simulink model "IEEE5BusSystemModel_std_UFLS"  (R2019b)
settings: Solver=ode4  StartTime=0.0  StopTime=300  MaxStep=1e-4  RelTol=1e-3
InitFcn:
  | startup_RTS
values from neighbouring files (symbols this model uses):
  C = b/(2*pi*60*Zn)    [startup_RTS.m]
  C0 = C/3    [startup_RTS.m]
  fn = 50    [startup_RTS.m]
  In = Sn/(sqrt(3)*Vn)    [startup_RTS.m]
  L = x*Zn/(2*pi*60)    [startup_RTS.m]
  L0 = 3*L    [startup_RTS.m]
  len = ceil(0.95*300000*T_prop)    [startup_RTS.m]
  PL1 = 300e6    (= 300000000)    [startup_RTS.m]
  PL2 = 300e6    (= 300000000)    [startup_RTS.m]
  PL3 = 300e6    (= 300000000)    [startup_RTS.m]
  QL1 = 30e6    (= 30000000)    [startup_RTS.m]
  QL2 = 30e6    (= 30000000)    [startup_RTS.m]
  QL3 = 30e6    (= 30000000)    [startup_RTS.m]
  R = r*Zn    [startup_RTS.m]
  R0 = 3*R    [startup_RTS.m]
  Sn = 1000e6    (= 1000000000)    [startup_RTS.m]
  t_cont = 100    [startup_RTS.m]
  Vn = 345e3    (= 345000)    [startup_RTS.m]
undefined symbols (not defined in the file or in its folder): D1, Delta
libraries: powerlib x42, powerlib_meascontrol x39, dspswit3 x10, dspstat3 x3, sps_avr x3, spsExcitationSystemModel x3
(part 2 of 7)

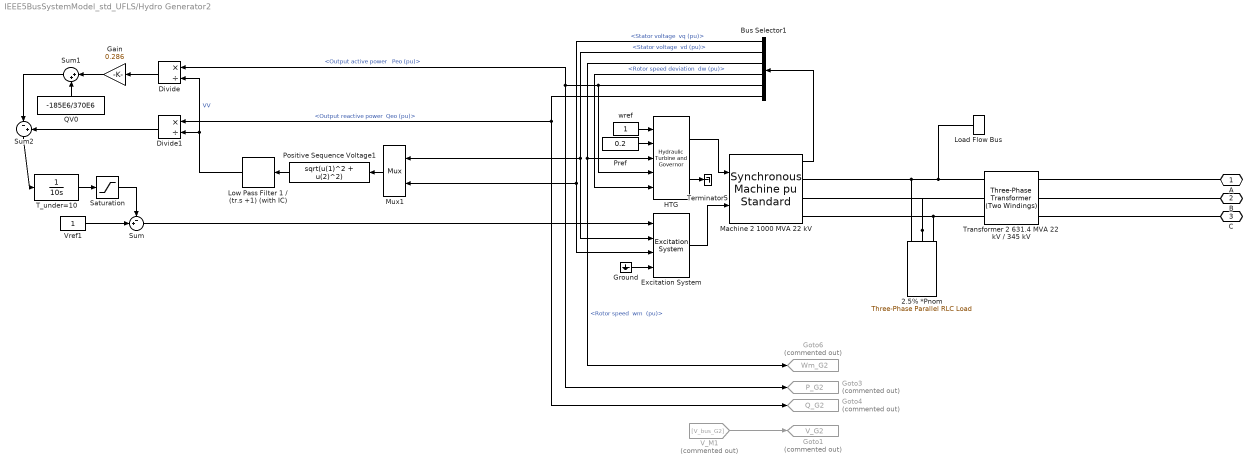
== system IEEE5BusSystemModel_std_UFLS/Hydro Generator2 ==
  2.5% *Pnom : powerlib/Elements/Three-Phase Parallel RLC Load  LConnTagsString=A|B|C  Configuration=Y (grounded)  NominalVoltage=vNom*1e3  Vabc=[1e3 1e3 1e3]  Vabcp=[1e3 1e3 1e3]  NominalFrequency=50  UnbalancedPower=off  ActivePower=pTotal*1e6*0.025  InductivePower=0  CapacitivePower=0  Pabc=[10e3 9e3 11e3]  QLabc=[100 90 110]  QCabc=[100 90 110]  Pabcp=[10e3 9e3 11e3]  QLabcp=[100 90 110]  QCabcp=[100 90 110]  Measurements=None  LoadType=constant Z
      settings: SourceProductName=Simscape Electrical
  Bus Selector1 : BusSelector  OutputSignals="dq0 components.Stator voltage  vq (pu),dq0 components.Stator voltage  vd (pu),Mechanical.Rotor speed  wm  (pu),Mechanical.Rotor speed deviation  dw (pu),Output active power   Peo (pu),Output reactive power  Qeo (pu)"
  Divide : Product  Inputs=*/
  Divide1 : Product  Inputs=*/
  Excitation System : sps_avr/Excitation System  tr=20e-3  reg=[ 200, 0.02 ]  exc=[ 1, 0 .19]  tgr=[ 0, 0 ]  damp=[ 0.0012, 1 ]  sat=[ 0, 0 ]  lim=[ 0, 7.32, 0 ]  v0=[1 1.0103]
      settings: SourceProductName=Simscape Electrical  SourceProductBaseCode=PS
  Gain : Gain  Gain=0.286
  Goto1 : Goto  Commented=on  GotoTag=V_G2  TagVisibility=global
  Goto3 : Goto  Commented=on  GotoTag=P_G2  TagVisibility=global
  Goto4 : Goto  Commented=on  GotoTag=Q_G2  TagVisibility=global
  Goto6 : Goto  Commented=on  GotoTag=Wm_G2  TagVisibility=global
  Ground : Ground
  HTG : powerlib/Machines/Hydraulic Turbine and Governor  sm="[ 10/3  0.07 ]"  gate="[  0.01  0.97518  -0.1  0.1 ]"  reg="[  0.05  1.163  0.105  0  0.01  ]"  hyd="[  0  2.67  ]"  dref=0  po=0.2002
      settings: SourceProductName=Simscape Electrical  SourceProductBaseCode=PS
  Load Flow Bus : powerlib/Measurements/Load Flow Bus  LConnTagsString=a  Phases=single  Connectors=on one side  ID=BUS_2_3  Vbase=22e3  Vref=1  Vangle=0  VLF=1  VLFb=1  VLFc=1  angleLF=-4.793  angleLFb=0  angleLFc=0
      settings: SourceProductName=Simscape Electrical
  Low Pass Filter 1 / (tr.s +1) (with IC) : spsExcitationSystemModel/Discrete/Low Pass Filter 1 // (tr.s +1) (with IC)  FilterType=Lowpass  Tc=20e-3  Ts=25e-6  Initialize=on  Vac_Init=[0 0 50]  Vdc_Init=1  PlotResponse=off  param1=[1 500 0.1]
      settings: SourceProductName=Simscape Electrical  SourceProductBaseCode=PS
  Machine 2 1000 MVA 22 kV : powerlib/Machines/Synchronous Machine pu Standard  PresetModel=No  MechanicalLoad=Mechanical power Pm  ShowDetailedParameters=on  RotorType=Round  Units=per unit standard parameters  MeasurementBus=off  NominalParameters=[pTotal*1e+006 vNom*1e3 fNom]  Reactances1=[ 1.693 0.4 0.2 1.618 0.967 0.2 0.035 ]  Reactances2=[1.699 0.174 0.109 0.838 0.185 0.069]  dAxisTimeConstants=Open-circuit  qAxisTimeConstants=Open-circuit  TimeConstants1=[]  TimeConstants2=[6.56 0.03 1.5 0.04]  TimeConstants3=[]  TimeConstants4=[]  TimeConstants5=[ 9.2, 0.01, 0.01 ]  TimeConstants6=[]  TimeConstants7=[0.024 0.006 0.006]  TimeConstants8=[1 2 3 1]  StatorResistance=0.005  Mechanical=[5.28 0.02558 2]  PolePairs=2  InitialConditions=[0 -76.0492 0.202092 0.202092 0.202092 3.45918 -116.541 123.459 1.01026]  SetSaturation=off  Saturation=[0.6404,0.7127,0.8441,0.9214,0.9956,1.082,1.19,1.316,1.457;0.7,0.7698,0.8872,0.9466,0.9969,1.046,1.1,1.151,1.201]  LoadFlowParameters=[1 524200000 21604 0]  TsPowergui=0  TsBlock=-1  IterativeModel=Trapezoidal non iterative  IterativeDiscreteModel=Trapezoidal non iterative  BusType=PV  Pref=200e6  Qref=0  Qmin=-100e6  Qmax=100e6  PLF=0  QLF=0
      settings: AttributesFormatString=\n\n  SourceProductName=Simscape Electrical
  Mux1 : Mux  Inputs=2
  Positive Sequence Voltage1 : Fcn  Expr=sqrt(u(1)^2 + u(2)^2)
  Pref : Constant  Value=0.2
  QV0 : Constant  Value=-185E6/370E6
  Saturation : Saturate  UpperLimit=0  LowerLimit=-10
  Sum : Sum  Inputs=-+|
  Sum1 : Sum  Inputs=|++
  Sum2 : Sum  Inputs=|-+
  T_under=10 : TransferFcn  Denominator=[10 0 ]
  Terminator5 : Terminator
  Transformer 2 631.4 MVA 22 kV / 345 kV : powerlib/Elements/Three-Phase Transformer (Two Windings)  Winding1Connection=Delta (D1)  Winding2Connection=Yg  CoreType=Three single-phase transformers  SetSaturation=off  Hysteresis=off  DataFile='hysteresis'  SetInitialFlux=off  Measurements=None  UNITS=pu  NominalPower=[ pTotal*1e+6 fNom ]  Winding1="[vNom*1e3   0.0     0.025*pTotal/100/2]"  Winding2="[ 1.07*345e3  0.0     0.025*pTotal/100/2 ]"  Rm=500  Lm=500  L0=0.5  Saturation="[ 0,0  ;  0.005,1.2  ;  1.0,1.4 ]"  InitialFluxes=[ 0.8 , -0.8 , 0.7 ]  BreakLoop=off  DiscreteSolver=Trapezoidal iterative  DataType=off  TransfoNumber=0
      settings: SourceProductName=Simscape Electrical
  V_M1 : From  Commented=on  GotoTag=V_bus_G2
  Vref1 : Constant
  wref : Constant
  A : PMIOPort  Side=Right
  B : PMIOPort  Port=2  Side=Right
  C : PMIOPort  Port=3  Side=Right
  wires:
  Ground/1 -> Excitation System/4
  HTG/2 -> Terminator5/1
  Sum/1 -> Excitation System/1
  Pref/1 -> HTG/2
  wref/1 -> HTG/1
  Excitation System/1 -> Machine 2 1000 MVA 22 kV/2
  HTG/1 -> Machine 2 1000 MVA 22 kV/1
  Machine 2 1000 MVA 22 kV/1 -> Bus Selector1/1
  Bus Selector1/3 -> HTG/3, Goto6/1  "<Rotor speed  wm  (pu)>"
  Bus Selector1/4 -> HTG/5  "<Rotor speed deviation  dw (pu)>"
  Bus Selector1/6 -> Divide1/1, Goto4/1  "<Output reactive power  Qeo (pu)>"
  V_M1/1 -> Goto1/1
  Saturation/1 -> Sum/1
  Gain/1 -> Sum1/1
  Sum1/1 -> Sum2/1
  Positive Sequence Voltage1/1 -> Low Pass Filter 1 / (tr.s +1) (with IC)/1
  Vref1/1 -> Sum/2
  Bus Selector1/5 -> HTG/4, Divide/1, Goto3/1  "<Output active power   Peo (pu)>"
  Divide/1 -> Gain/1
  Low Pass Filter 1 / (tr.s +1) (with IC)/1 -> Divide1/2, Divide/2  "VV"
  QV0/1 -> Sum1/2
  Sum2/1 -> T_under=10/1
  T_under=10/1 -> Saturation/1
  Mux1/1 -> Positive Sequence Voltage1/1
  Divide1/1 -> Sum2/2
  Bus Selector1/1 -> Mux1/2, Excitation System/3  "<Stator voltage  vq (pu)>"
  Bus Selector1/2 -> Mux1/1, Excitation System/2  "<Stator voltage  vd (pu)>"
  connections:
  C/RConn1 -- Transformer 2 631.4 MVA 22 kV / 345 kV/RConn3
  Transformer 2 631.4 MVA 22 kV / 345 kV/LConn1 -- Load Flow Bus/LConn1 -- Machine 2 1000 MVA 22 kV/RConn1 -- 2.5% *Pnom/LConn1
  2.5% *Pnom/LConn2 -- Transformer 2 631.4 MVA 22 kV / 345 kV/LConn2 -- Machine 2 1000 MVA 22 kV/RConn2
  A/RConn1 -- Transformer 2 631.4 MVA 22 kV / 345 kV/RConn1
  B/RConn1 -- Transformer 2 631.4 MVA 22 kV / 345 kV/RConn2
  Machine 2 1000 MVA 22 kV/RConn3 -- Transformer 2 631.4 MVA 22 kV / 345 kV/LConn3 -- 2.5% *Pnom/LConn3

== system IEEE5BusSystemModel_std_UFLS/Subsystem ==
  f1 : Inport
  f2 : Inport  Port=2
  f3 : Inport  Port=3
  Enable : EnablePort  PropagateVarSize=During execution
  Gain : Gain  Gain=fn
  Gain1 : Gain  Gain=fn
  Gain2 : Gain  Gain=fn
  loadshedding : Subsystem  TreatAsAtomicUnit=on  SystemSampleTime=0.0025
  loadshedding1 : Subsystem  TreatAsAtomicUnit=on  SystemSampleTime=0.0025
  loadshedding2 : Subsystem  TreatAsAtomicUnit=on  SystemSampleTime=0.0025
  Shedding factor 1 : Outport  VectorParamsAs1DForOutWhenUnconnected=off
  Shedding factor 2 : Outport  Port=2  VectorParamsAs1DForOutWhenUnconnected=off
  Shedding factor 3 : Outport  Port=3  VectorParamsAs1DForOutWhenUnconnected=off
  wires:
  Gain2/1 -> loadshedding2/1(Freq)
  loadshedding/1(Shedding factor) -> Shedding factor 1/1
  f1/1 -> Gain/1
  f3/1 -> Gain2/1
  Gain/1 -> loadshedding/1(Freq)
  Gain1/1 -> loadshedding1/1(Freq)
  f2/1 -> Gain1/1
  loadshedding1/1(Shedding factor) -> Shedding factor 2/1
  loadshedding2/1(Shedding factor) -> Shedding factor 3/1

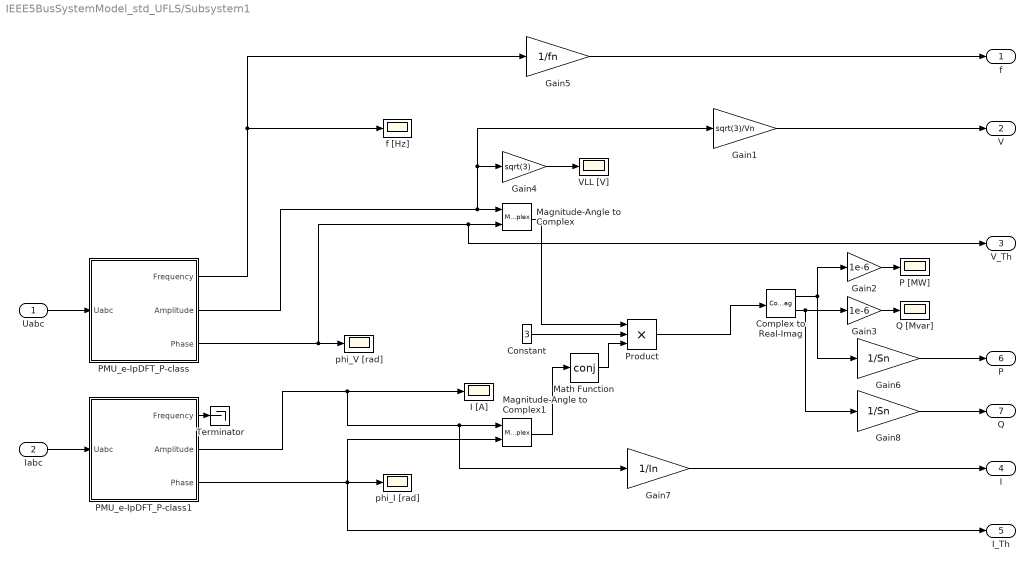
== system IEEE5BusSystemModel_std_UFLS/Subsystem1 ==
  Uabc : Inport  OutDataTypeStr=double  PortDimensions=3  SampleTime=[5.0000000000000002e-05,0]
  Iabc : Inport  Port=2  OutDataTypeStr=double  PortDimensions=3  SampleTime=[5.0000000000000002e-05,0]
  Complex to Real-Imag : ComplexToRealImag
  Constant : Constant  Value=3
  Gain1 : Gain  Gain=sqrt(3)/Vn
  Gain2 : Gain  Gain=1e-6
  Gain3 : Gain  Gain=1e-6
  Gain4 : Gain  Gain=sqrt(3)
  Gain5 : Gain  Gain=1/fn
  Gain6 : Gain  Gain=1/Sn
  Gain7 : Gain  Gain=1/In
  Gain8 : Gain  Gain=1/Sn
  I [A] : Scope
  Magnitude-Angle to Complex : MagnitudeAngleToComplex
  Magnitude-Angle to Complex1 : MagnitudeAngleToComplex
  Math Function : Math  Operator=conj  SaturateOnIntegerOverflow=on
  P [MW] : Scope
  PMU_e-IpDFT_P-class : Subsystem  TreatAsAtomicUnit=on  SystemSampleTime=100e-6  mask{f0=50, Fr=50, Fs=1e4, T=0.06, enable_comp=off, TdF=10}
      mask prompts: f0 "Nominal frequency (Hz)"; Fr "Data reporting rate (frames/s)"; Fs "Sampling rate (Hz)"; T "Window length (s)"; enable_comp "Compensate clock drift"; TdF "Clock drift measurement window length (s)"
      mask init:
      | dF = 1/T;
      | M = round(T*Fs);
      | kmax = round (f0*T);
      | k = kmax-2:kmax+2;
      | Wk = exp(-1i*2*pi*k./M);
      | Tr = 1/Fr;
      | Ts_p=1/Fs;
      mask DialogControl ParameterTabVar0 Prompt: Settings
  PMU_e-IpDFT_P-class1 : Subsystem  TreatAsAtomicUnit=on  SystemSampleTime=100e-6  mask{f0=50, Fr=50, Fs=1e4, T=0.06, enable_comp=off, TdF=10}
      mask prompts: f0 "Nominal frequency (Hz)"; Fr "Data reporting rate (frames/s)"; Fs "Sampling rate (Hz)"; T "Window length (s)"; enable_comp "Compensate clock drift"; TdF "Clock drift measurement window length (s)"
      mask init:
      | dF = 1/T;
      | M = round(T*Fs);
      | kmax = round (f0*T);
      | k = kmax-2:kmax+2;
      | Wk = exp(-1i*2*pi*k./M);
      | Tr = 1/Fr;
      | Ts_p=1/Fs;
      mask DialogControl ParameterTabVar0 Prompt: Settings
  Product : Product  Inputs=3
  Q [Mvar] : Scope
  Terminator : Terminator
  VLL [V] : Scope
  f [Hz] : Scope
  phi_I [rad] : Scope
  phi_V [rad] : Scope
  f : Outport  OutDataTypeStr=double  PortDimensions=1  SampleTime=[0.02,0]  VectorParamsAs1DForOutWhenUnconnected=off
  V : Outport  Port=2  OutDataTypeStr=double  PortDimensions=1  SampleTime=[0.02,0]  VectorParamsAs1DForOutWhenUnconnected=off
  V_Th : Outport  Port=3  OutDataTypeStr=double  PortDimensions=1  SampleTime=[0.02,0]  VectorParamsAs1DForOutWhenUnconnected=off
  I : Outport  Port=4  OutDataTypeStr=double  PortDimensions=1  SampleTime=[0.02,0]  VectorParamsAs1DForOutWhenUnconnected=off
  I_Th : Outport  Port=5  OutDataTypeStr=double  PortDimensions=1  SampleTime=[0.02,0]  VectorParamsAs1DForOutWhenUnconnected=off
  P : Outport  Port=6  OutDataTypeStr=double  PortDimensions=1  SampleTime=[0.02,0]  VectorParamsAs1DForOutWhenUnconnected=off
  Q : Outport  Port=7  OutDataTypeStr=double  PortDimensions=1  SampleTime=[0.02,0]  VectorParamsAs1DForOutWhenUnconnected=off
  wires:
  Gain8/1 -> Q/1
  Gain7/1 -> I/1
  Gain5/1 -> f/1
  Gain6/1 -> P/1
  Complex to Real-Imag/2 -> Gain3/1, Gain8/1
  Complex to Real-Imag/1 -> Gain2/1, Gain6/1
  Product/1 -> Complex to Real-Imag/1
  Math Function/1 -> Product/3
  Constant/1 -> Product/2
  Magnitude-Angle to Complex1/1 -> Math Function/1
  Gain1/1 -> V/1
  Magnitude-Angle to Complex/1 -> Product/1
  PMU_e-IpDFT_P-class1/1(Frequency) -> Terminator/1
  Gain4/1 -> VLL [V]/1
  Gain3/1 -> Q [Mvar]/1
  Uabc/1 -> PMU_e-IpDFT_P-class/1(Uabc)
  PMU_e-IpDFT_P-class1/2(Amplitude) -> I [A]/1, Magnitude-Angle to Complex1/1, Gain7/1
  PMU_e-IpDFT_P-class1/3(Phase) -> Magnitude-Angle to Complex1/2, phi_I [rad]/1, I_Th/1
  Gain2/1 -> P [MW]/1
  PMU_e-IpDFT_P-class/1(Frequency) -> f [Hz]/1, Gain5/1
  PMU_e-IpDFT_P-class/2(Amplitude) -> Magnitude-Angle to Complex/1, Gain4/1, Gain1/1
  PMU_e-IpDFT_P-class/3(Phase) -> Magnitude-Angle to Complex/2, V_Th/1, phi_V [rad]/1
  Iabc/1 -> PMU_e-IpDFT_P-class1/1(Uabc)

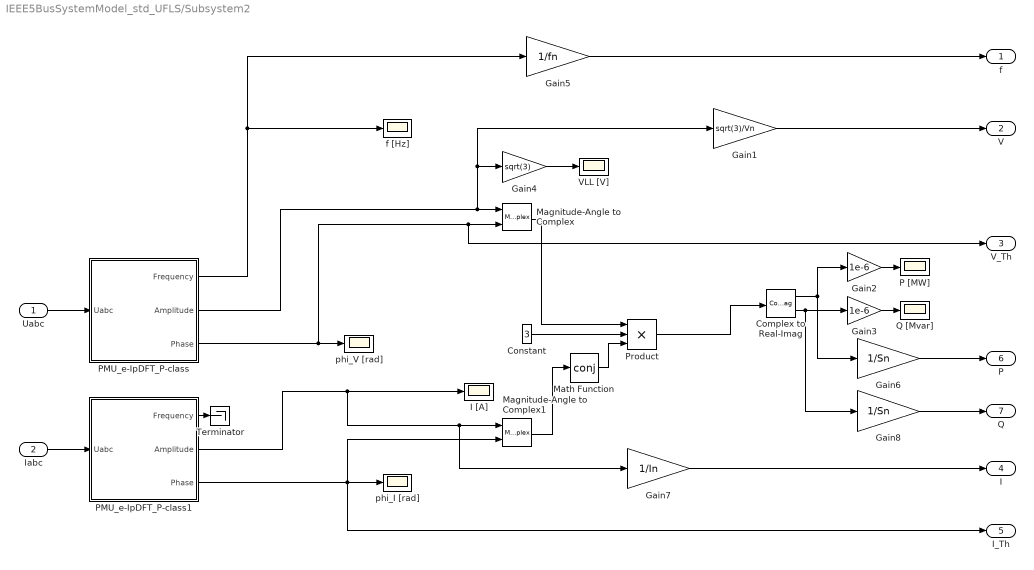
== system IEEE5BusSystemModel_std_UFLS/Subsystem2 ==
  Uabc : Inport  OutDataTypeStr=double  PortDimensions=3  SampleTime=[5.0000000000000002e-05,0]
  Iabc : Inport  Port=2  OutDataTypeStr=double  PortDimensions=3  SampleTime=[5.0000000000000002e-05,0]
  Complex to Real-Imag : ComplexToRealImag
  Constant : Constant  Value=3
  Gain1 : Gain  Gain=sqrt(3)/Vn
  Gain2 : Gain  Gain=1e-6
  Gain3 : Gain  Gain=1e-6
  Gain4 : Gain  Gain=sqrt(3)
  Gain5 : Gain  Gain=1/fn
  Gain6 : Gain  Gain=1/Sn
  Gain7 : Gain  Gain=1/In
  Gain8 : Gain  Gain=1/Sn
  I [A] : Scope
  Magnitude-Angle to Complex : MagnitudeAngleToComplex
  Magnitude-Angle to Complex1 : MagnitudeAngleToComplex
  Math Function : Math  Operator=conj  SaturateOnIntegerOverflow=on
  P [MW] : Scope
  PMU_e-IpDFT_P-class : Subsystem  TreatAsAtomicUnit=on  SystemSampleTime=100e-6  mask{f0=50, Fr=50, Fs=1e4, T=0.06, enable_comp=off, TdF=10}
      mask prompts: f0 "Nominal frequency (Hz)"; Fr "Data reporting rate (frames/s)"; Fs "Sampling rate (Hz)"; T "Window length (s)"; enable_comp "Compensate clock drift"; TdF "Clock drift measurement window length (s)"
      mask init:
      | dF = 1/T;
      | M = round(T*Fs);
      | kmax = round (f0*T);
      | k = kmax-2:kmax+2;
      | Wk = exp(-1i*2*pi*k./M);
      | Tr = 1/Fr;
      | Ts_p=1/Fs;
      mask DialogControl ParameterTabVar0 Prompt: Settings
  PMU_e-IpDFT_P-class1 : Subsystem  TreatAsAtomicUnit=on  SystemSampleTime=100e-6  mask{f0=50, Fr=50, Fs=1e4, T=0.06, enable_comp=off, TdF=10}
      mask prompts: f0 "Nominal frequency (Hz)"; Fr "Data reporting rate (frames/s)"; Fs "Sampling rate (Hz)"; T "Window length (s)"; enable_comp "Compensate clock drift"; TdF "Clock drift measurement window length (s)"
      mask init:
      | dF = 1/T;
      | M = round(T*Fs);
      | kmax = round (f0*T);
      | k = kmax-2:kmax+2;
      | Wk = exp(-1i*2*pi*k./M);
      | Tr = 1/Fr;
      | Ts_p=1/Fs;
      mask DialogControl ParameterTabVar0 Prompt: Settings
  Product : Product  Inputs=3
  Q [Mvar] : Scope
  Terminator : Terminator
  VLL [V] : Scope
  f [Hz] : Scope
  phi_I [rad] : Scope
  phi_V [rad] : Scope
  f : Outport  OutDataTypeStr=double  PortDimensions=1  SampleTime=[0.02,0]  VectorParamsAs1DForOutWhenUnconnected=off
  V : Outport  Port=2  OutDataTypeStr=double  PortDimensions=1  SampleTime=[0.02,0]  VectorParamsAs1DForOutWhenUnconnected=off
  V_Th : Outport  Port=3  OutDataTypeStr=double  PortDimensions=1  SampleTime=[0.02,0]  VectorParamsAs1DForOutWhenUnconnected=off
  I : Outport  Port=4  OutDataTypeStr=double  PortDimensions=1  SampleTime=[0.02,0]  VectorParamsAs1DForOutWhenUnconnected=off
  I_Th : Outport  Port=5  OutDataTypeStr=double  PortDimensions=1  SampleTime=[0.02,0]  VectorParamsAs1DForOutWhenUnconnected=off
  P : Outport  Port=6  OutDataTypeStr=double  PortDimensions=1  SampleTime=[0.02,0]  VectorParamsAs1DForOutWhenUnconnected=off
  Q : Outport  Port=7  OutDataTypeStr=double  PortDimensions=1  SampleTime=[0.02,0]  VectorParamsAs1DForOutWhenUnconnected=off
  wires:
  Iabc/1 -> PMU_e-IpDFT_P-class1/1(Uabc)
  PMU_e-IpDFT_P-class/3(Phase) -> phi_V [rad]/1, V_Th/1, Magnitude-Angle to Complex/2
  PMU_e-IpDFT_P-class/2(Amplitude) -> Gain1/1, Gain4/1, Magnitude-Angle to Complex/1
  PMU_e-IpDFT_P-class/1(Frequency) -> Gain5/1, f [Hz]/1
  Gain2/1 -> P [MW]/1
  PMU_e-IpDFT_P-class1/3(Phase) -> I_Th/1, phi_I [rad]/1, Magnitude-Angle to Complex1/2
  PMU_e-IpDFT_P-class1/2(Amplitude) -> Gain7/1, Magnitude-Angle to Complex1/1, I [A]/1
  Uabc/1 -> PMU_e-IpDFT_P-class/1(Uabc)
  Gain3/1 -> Q [Mvar]/1
  Gain4/1 -> VLL [V]/1
  PMU_e-IpDFT_P-class1/1(Frequency) -> Terminator/1
  Magnitude-Angle to Complex/1 -> Product/1
  Gain1/1 -> V/1
  Magnitude-Angle to Complex1/1 -> Math Function/1
  Constant/1 -> Product/2
  Math Function/1 -> Product/3
  Product/1 -> Complex to Real-Imag/1
  Complex to Real-Imag/1 -> Gain6/1, Gain2/1
  Complex to Real-Imag/2 -> Gain8/1, Gain3/1
  Gain6/1 -> P/1
  Gain5/1 -> f/1
  Gain7/1 -> I/1
  Gain8/1 -> Q/1

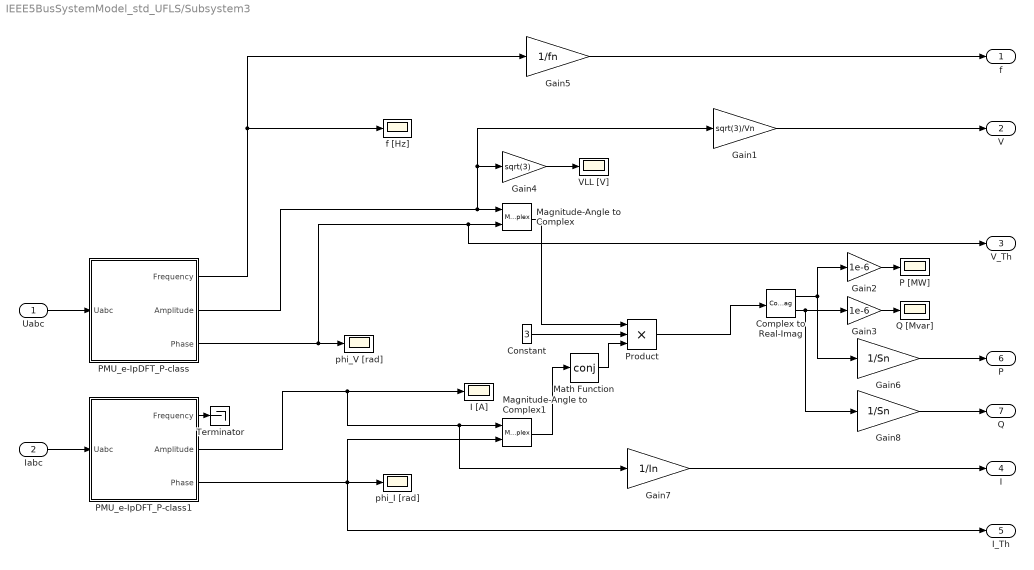
== system IEEE5BusSystemModel_std_UFLS/Subsystem3 ==
  Uabc : Inport  OutDataTypeStr=double  PortDimensions=3  SampleTime=[5.0000000000000002e-05,0]
  Iabc : Inport  Port=2  OutDataTypeStr=double  PortDimensions=3  SampleTime=[5.0000000000000002e-05,0]
  Complex to Real-Imag : ComplexToRealImag
  Constant : Constant  Value=3
  Gain1 : Gain  Gain=sqrt(3)/Vn
  Gain2 : Gain  Gain=1e-6
  Gain3 : Gain  Gain=1e-6
  Gain4 : Gain  Gain=sqrt(3)
  Gain5 : Gain  Gain=1/fn
  Gain6 : Gain  Gain=1/Sn
  Gain7 : Gain  Gain=1/In
  Gain8 : Gain  Gain=1/Sn
  I [A] : Scope
  Magnitude-Angle to Complex : MagnitudeAngleToComplex
  Magnitude-Angle to Complex1 : MagnitudeAngleToComplex
  Math Function : Math  Operator=conj  SaturateOnIntegerOverflow=on
  P [MW] : Scope
  PMU_e-IpDFT_P-class : Subsystem  TreatAsAtomicUnit=on  SystemSampleTime=100e-6  mask{f0=50, Fr=50, Fs=1e4, T=0.06, enable_comp=off, TdF=10}
      mask prompts: f0 "Nominal frequency (Hz)"; Fr "Data reporting rate (frames/s)"; Fs "Sampling rate (Hz)"; T "Window length (s)"; enable_comp "Compensate clock drift"; TdF "Clock drift measurement window length (s)"
      mask init:
      | dF = 1/T;
      | M = round(T*Fs);
      | kmax = round (f0*T);
      | k = kmax-2:kmax+2;
      | Wk = exp(-1i*2*pi*k./M);
      | Tr = 1/Fr;
      | Ts_p=1/Fs;
      mask DialogControl ParameterTabVar0 Prompt: Settings
  PMU_e-IpDFT_P-class1 : Subsystem  TreatAsAtomicUnit=on  SystemSampleTime=100e-6  mask{f0=50, Fr=50, Fs=1e4, T=0.06, enable_comp=off, TdF=10}
      mask prompts: f0 "Nominal frequency (Hz)"; Fr "Data reporting rate (frames/s)"; Fs "Sampling rate (Hz)"; T "Window length (s)"; enable_comp "Compensate clock drift"; TdF "Clock drift measurement window length (s)"
      mask init:
      | dF = 1/T;
      | M = round(T*Fs);
      | kmax = round (f0*T);
      | k = kmax-2:kmax+2;
      | Wk = exp(-1i*2*pi*k./M);
      | Tr = 1/Fr;
      | Ts_p=1/Fs;
      mask DialogControl ParameterTabVar0 Prompt: Settings
  Product : Product  Inputs=3
  Q [Mvar] : Scope
  Terminator : Terminator
  VLL [V] : Scope
  f [Hz] : Scope
  phi_I [rad] : Scope
  phi_V [rad] : Scope
  f : Outport  OutDataTypeStr=double  PortDimensions=1  SampleTime=[0.02,0]  VectorParamsAs1DForOutWhenUnconnected=off
  V : Outport  Port=2  OutDataTypeStr=double  PortDimensions=1  SampleTime=[0.02,0]  VectorParamsAs1DForOutWhenUnconnected=off
  V_Th : Outport  Port=3  OutDataTypeStr=double  PortDimensions=1  SampleTime=[0.02,0]  VectorParamsAs1DForOutWhenUnconnected=off
  I : Outport  Port=4  OutDataTypeStr=double  PortDimensions=1  SampleTime=[0.02,0]  VectorParamsAs1DForOutWhenUnconnected=off
  I_Th : Outport  Port=5  OutDataTypeStr=double  PortDimensions=1  SampleTime=[0.02,0]  VectorParamsAs1DForOutWhenUnconnected=off
  P : Outport  Port=6  OutDataTypeStr=double  PortDimensions=1  SampleTime=[0.02,0]  VectorParamsAs1DForOutWhenUnconnected=off
  Q : Outport  Port=7  OutDataTypeStr=double  PortDimensions=1  SampleTime=[0.02,0]  VectorParamsAs1DForOutWhenUnconnected=off
  wires:
  Gain8/1 -> Q/1
  Gain7/1 -> I/1
  Gain5/1 -> f/1
  Gain6/1 -> P/1
  Complex to Real-Imag/2 -> Gain3/1, Gain8/1
  Complex to Real-Imag/1 -> Gain2/1, Gain6/1
  Product/1 -> Complex to Real-Imag/1
  Math Function/1 -> Product/3
  Constant/1 -> Product/2
  Magnitude-Angle to Complex1/1 -> Math Function/1
  Gain1/1 -> V/1
  Magnitude-Angle to Complex/1 -> Product/1
  PMU_e-IpDFT_P-class1/1(Frequency) -> Terminator/1
  Gain4/1 -> VLL [V]/1
  Gain3/1 -> Q [Mvar]/1
  Uabc/1 -> PMU_e-IpDFT_P-class/1(Uabc)
  PMU_e-IpDFT_P-class1/2(Amplitude) -> I [A]/1, Magnitude-Angle to Complex1/1, Gain7/1
  PMU_e-IpDFT_P-class1/3(Phase) -> Magnitude-Angle to Complex1/2, phi_I [rad]/1, I_Th/1
  Gain2/1 -> P [MW]/1
  PMU_e-IpDFT_P-class/1(Frequency) -> f [Hz]/1, Gain5/1
  PMU_e-IpDFT_P-class/2(Amplitude) -> Magnitude-Angle to Complex/1, Gain4/1, Gain1/1
  PMU_e-IpDFT_P-class/3(Phase) -> Magnitude-Angle to Complex/2, V_Th/1, phi_V [rad]/1
  Iabc/1 -> PMU_e-IpDFT_P-class1/1(Uabc)

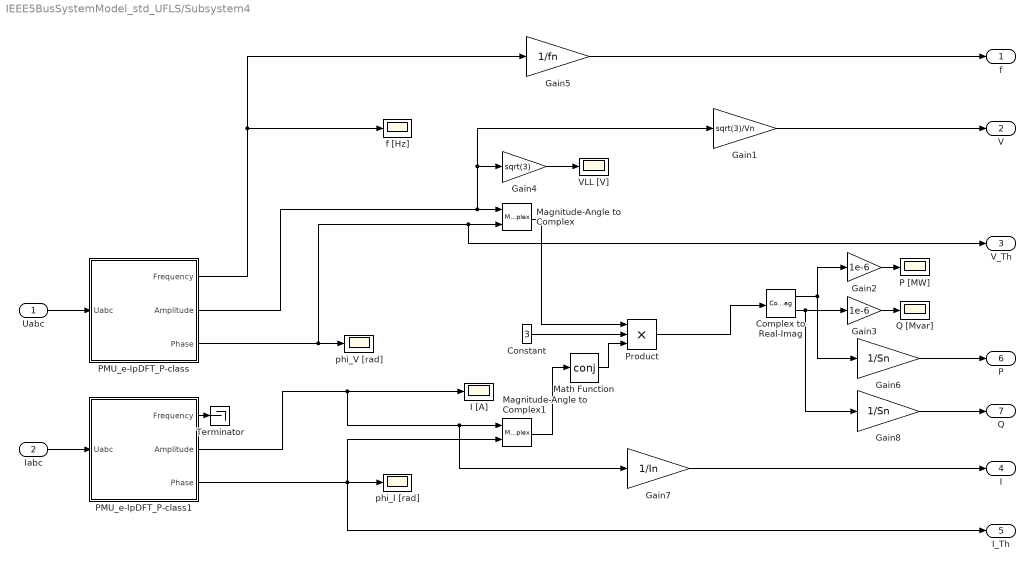
== system IEEE5BusSystemModel_std_UFLS/Subsystem4 ==
  Uabc : Inport  OutDataTypeStr=double  PortDimensions=3  SampleTime=[5.0000000000000002e-05,0]
  Iabc : Inport  Port=2  OutDataTypeStr=double  PortDimensions=3  SampleTime=[5.0000000000000002e-05,0]
  Complex to Real-Imag : ComplexToRealImag
  Constant : Constant  Value=3
  Gain1 : Gain  Gain=sqrt(3)/Vn
  Gain2 : Gain  Gain=1e-6
  Gain3 : Gain  Gain=1e-6
  Gain4 : Gain  Gain=sqrt(3)
  Gain5 : Gain  Gain=1/fn
  Gain6 : Gain  Gain=1/Sn
  Gain7 : Gain  Gain=1/In
  Gain8 : Gain  Gain=1/Sn
  I [A] : Scope
  Magnitude-Angle to Complex : MagnitudeAngleToComplex
  Magnitude-Angle to Complex1 : MagnitudeAngleToComplex
  Math Function : Math  Operator=conj  SaturateOnIntegerOverflow=on
  P [MW] : Scope
  PMU_e-IpDFT_P-class : Subsystem  TreatAsAtomicUnit=on  SystemSampleTime=100e-6  mask{f0=50, Fr=50, Fs=1e4, T=0.06, enable_comp=off, TdF=10}
      mask prompts: f0 "Nominal frequency (Hz)"; Fr "Data reporting rate (frames/s)"; Fs "Sampling rate (Hz)"; T "Window length (s)"; enable_comp "Compensate clock drift"; TdF "Clock drift measurement window length (s)"
      mask init:
      | dF = 1/T;
      | M = round(T*Fs);
      | kmax = round (f0*T);
      | k = kmax-2:kmax+2;
      | Wk = exp(-1i*2*pi*k./M);
      | Tr = 1/Fr;
      | Ts_p=1/Fs;
      mask DialogControl ParameterTabVar0 Prompt: Settings
  PMU_e-IpDFT_P-class1 : Subsystem  TreatAsAtomicUnit=on  SystemSampleTime=100e-6  mask{f0=50, Fr=50, Fs=1e4, T=0.06, enable_comp=off, TdF=10}
      mask prompts: f0 "Nominal frequency (Hz)"; Fr "Data reporting rate (frames/s)"; Fs "Sampling rate (Hz)"; T "Window length (s)"; enable_comp "Compensate clock drift"; TdF "Clock drift measurement window length (s)"
      mask init:
      | dF = 1/T;
      | M = round(T*Fs);
      | kmax = round (f0*T);
      | k = kmax-2:kmax+2;
      | Wk = exp(-1i*2*pi*k./M);
      | Tr = 1/Fr;
      | Ts_p=1/Fs;
      mask DialogControl ParameterTabVar0 Prompt: Settings
  Product : Product  Inputs=3
  Q [Mvar] : Scope
  Terminator : Terminator
  VLL [V] : Scope
  f [Hz] : Scope
  phi_I [rad] : Scope
  phi_V [rad] : Scope
  f : Outport  OutDataTypeStr=double  PortDimensions=1  SampleTime=[0.02,0]  VectorParamsAs1DForOutWhenUnconnected=off
  V : Outport  Port=2  OutDataTypeStr=double  PortDimensions=1  SampleTime=[0.02,0]  VectorParamsAs1DForOutWhenUnconnected=off
  V_Th : Outport  Port=3  OutDataTypeStr=double  PortDimensions=1  SampleTime=[0.02,0]  VectorParamsAs1DForOutWhenUnconnected=off
  I : Outport  Port=4  OutDataTypeStr=double  PortDimensions=1  SampleTime=[0.02,0]  VectorParamsAs1DForOutWhenUnconnected=off
  I_Th : Outport  Port=5  OutDataTypeStr=double  PortDimensions=1  SampleTime=[0.02,0]  VectorParamsAs1DForOutWhenUnconnected=off
  P : Outport  Port=6  OutDataTypeStr=double  PortDimensions=1  SampleTime=[0.02,0]  VectorParamsAs1DForOutWhenUnconnected=off
  Q : Outport  Port=7  OutDataTypeStr=double  PortDimensions=1  SampleTime=[0.02,0]  VectorParamsAs1DForOutWhenUnconnected=off
  wires:
  Iabc/1 -> PMU_e-IpDFT_P-class1/1(Uabc)
  PMU_e-IpDFT_P-class/3(Phase) -> phi_V [rad]/1, V_Th/1, Magnitude-Angle to Complex/2
  PMU_e-IpDFT_P-class/2(Amplitude) -> Gain1/1, Gain4/1, Magnitude-Angle to Complex/1
  PMU_e-IpDFT_P-class/1(Frequency) -> Gain5/1, f [Hz]/1
  Gain2/1 -> P [MW]/1
  PMU_e-IpDFT_P-class1/3(Phase) -> I_Th/1, phi_I [rad]/1, Magnitude-Angle to Complex1/2
  PMU_e-IpDFT_P-class1/2(Amplitude) -> Gain7/1, Magnitude-Angle to Complex1/1, I [A]/1
  Uabc/1 -> PMU_e-IpDFT_P-class/1(Uabc)
  Gain3/1 -> Q [Mvar]/1
  Gain4/1 -> VLL [V]/1
  PMU_e-IpDFT_P-class1/1(Frequency) -> Terminator/1
  Magnitude-Angle to Complex/1 -> Product/1
  Gain1/1 -> V/1
  Magnitude-Angle to Complex1/1 -> Math Function/1
  Constant/1 -> Product/2
  Math Function/1 -> Product/3
  Product/1 -> Complex to Real-Imag/1
  Complex to Real-Imag/1 -> Gain6/1, Gain2/1
  Complex to Real-Imag/2 -> Gain8/1, Gain3/1
  Gain6/1 -> P/1
  Gain5/1 -> f/1
  Gain7/1 -> I/1
  Gain8/1 -> Q/1

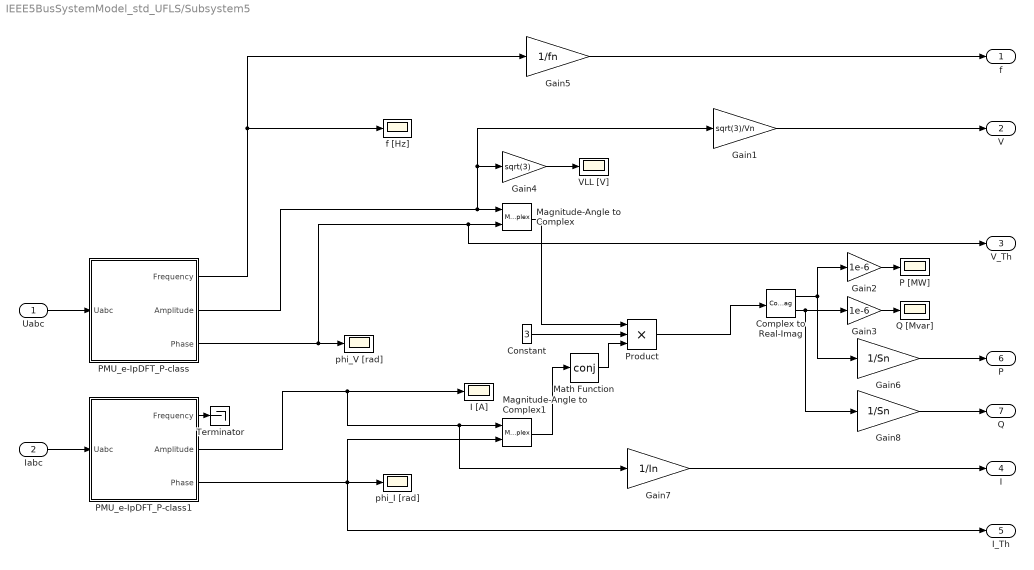
== system IEEE5BusSystemModel_std_UFLS/Subsystem5 ==
  Uabc : Inport  OutDataTypeStr=double  PortDimensions=3  SampleTime=[5.0000000000000002e-05,0]
  Iabc : Inport  Port=2  OutDataTypeStr=double  PortDimensions=3  SampleTime=[5.0000000000000002e-05,0]
  Complex to Real-Imag : ComplexToRealImag
  Constant : Constant  Value=3
  Gain1 : Gain  Gain=sqrt(3)/Vn
  Gain2 : Gain  Gain=1e-6
  Gain3 : Gain  Gain=1e-6
  Gain4 : Gain  Gain=sqrt(3)
  Gain5 : Gain  Gain=1/fn
  Gain6 : Gain  Gain=1/Sn
  Gain7 : Gain  Gain=1/In
  Gain8 : Gain  Gain=1/Sn
  I [A] : Scope
  Magnitude-Angle to Complex : MagnitudeAngleToComplex
  Magnitude-Angle to Complex1 : MagnitudeAngleToComplex
  Math Function : Math  Operator=conj  SaturateOnIntegerOverflow=on
  P [MW] : Scope
  PMU_e-IpDFT_P-class : Subsystem  TreatAsAtomicUnit=on  SystemSampleTime=100e-6  mask{f0=50, Fr=50, Fs=1e4, T=0.06, enable_comp=off, TdF=10}
      mask prompts: f0 "Nominal frequency (Hz)"; Fr "Data reporting rate (frames/s)"; Fs "Sampling rate (Hz)"; T "Window length (s)"; enable_comp "Compensate clock drift"; TdF "Clock drift measurement window length (s)"
      mask init:
      | dF = 1/T;
      | M = round(T*Fs);
      | kmax = round (f0*T);
      | k = kmax-2:kmax+2;
      | Wk = exp(-1i*2*pi*k./M);
      | Tr = 1/Fr;
      | Ts_p=1/Fs;
      mask DialogControl ParameterTabVar0 Prompt: Settings
  PMU_e-IpDFT_P-class1 : Subsystem  TreatAsAtomicUnit=on  SystemSampleTime=100e-6  mask{f0=50, Fr=50, Fs=1e4, T=0.06, enable_comp=off, TdF=10}
      mask prompts: f0 "Nominal frequency (Hz)"; Fr "Data reporting rate (frames/s)"; Fs "Sampling rate (Hz)"; T "Window length (s)"; enable_comp "Compensate clock drift"; TdF "Clock drift measurement window length (s)"
      mask init:
      | dF = 1/T;
      | M = round(T*Fs);
      | kmax = round (f0*T);
      | k = kmax-2:kmax+2;
      | Wk = exp(-1i*2*pi*k./M);
      | Tr = 1/Fr;
      | Ts_p=1/Fs;
      mask DialogControl ParameterTabVar0 Prompt: Settings
  Product : Product  Inputs=3
  Q [Mvar] : Scope
  Terminator : Terminator
  VLL [V] : Scope
  f [Hz] : Scope
  phi_I [rad] : Scope
  phi_V [rad] : Scope
  f : Outport  OutDataTypeStr=double  PortDimensions=1  SampleTime=[0.02,0]  VectorParamsAs1DForOutWhenUnconnected=off
  V : Outport  Port=2  OutDataTypeStr=double  PortDimensions=1  SampleTime=[0.02,0]  VectorParamsAs1DForOutWhenUnconnected=off
  V_Th : Outport  Port=3  OutDataTypeStr=double  PortDimensions=1  SampleTime=[0.02,0]  VectorParamsAs1DForOutWhenUnconnected=off
  I : Outport  Port=4  OutDataTypeStr=double  PortDimensions=1  SampleTime=[0.02,0]  VectorParamsAs1DForOutWhenUnconnected=off
  I_Th : Outport  Port=5  OutDataTypeStr=double  PortDimensions=1  SampleTime=[0.02,0]  VectorParamsAs1DForOutWhenUnconnected=off
  P : Outport  Port=6  OutDataTypeStr=double  PortDimensions=1  SampleTime=[0.02,0]  VectorParamsAs1DForOutWhenUnconnected=off
  Q : Outport  Port=7  OutDataTypeStr=double  PortDimensions=1  SampleTime=[0.02,0]  VectorParamsAs1DForOutWhenUnconnected=off
  wires:
  Iabc/1 -> PMU_e-IpDFT_P-class1/1(Uabc)
  PMU_e-IpDFT_P-class/3(Phase) -> phi_V [rad]/1, V_Th/1, Magnitude-Angle to Complex/2
  PMU_e-IpDFT_P-class/2(Amplitude) -> Gain1/1, Gain4/1, Magnitude-Angle to Complex/1
  PMU_e-IpDFT_P-class/1(Frequency) -> Gain5/1, f [Hz]/1
  Gain2/1 -> P [MW]/1
  PMU_e-IpDFT_P-class1/3(Phase) -> I_Th/1, phi_I [rad]/1, Magnitude-Angle to Complex1/2
  PMU_e-IpDFT_P-class1/2(Amplitude) -> Gain7/1, Magnitude-Angle to Complex1/1, I [A]/1
  Uabc/1 -> PMU_e-IpDFT_P-class/1(Uabc)
  Gain3/1 -> Q [Mvar]/1
  Gain4/1 -> VLL [V]/1
  PMU_e-IpDFT_P-class1/1(Frequency) -> Terminator/1
  Magnitude-Angle to Complex/1 -> Product/1
  Gain1/1 -> V/1
  Magnitude-Angle to Complex1/1 -> Math Function/1
  Constant/1 -> Product/2
  Math Function/1 -> Product/3
  Product/1 -> Complex to Real-Imag/1
  Complex to Real-Imag/1 -> Gain6/1, Gain2/1
  Complex to Real-Imag/2 -> Gain8/1, Gain3/1
  Gain6/1 -> P/1
  Gain5/1 -> f/1
  Gain7/1 -> I/1
  Gain8/1 -> Q/1

== system IEEE5BusSystemModel_std_UFLS/Dynamic Load/Load 8 ==
  note: 200ms buffer for average voltag and frequency
      | to avoid oscillation
  Vabc : Inport
  "[P0,Q0]" : Inport  Port=2
  Buffer1 : Buffer  N=2400  V=2200
  Buffer2 : Buffer  N=240  V=220
  Demux : Demux  Outputs=[1 1 1]
  Gain : Gain  Gain=1/240
  Load shedding : Subsystem  TreatAsAtomicUnit=on  SystemSampleTime=20e-3
  PLL : powerlib_meascontrol/PLL/PLL  Fmin=45  Par_Init=[0, 50]  ParK=[180, 3200, 1]  TcD=1e-3  MaxRateChangeFreq=25  FilterCutOffFreq=25  Ts=1000e-6  AGC=on
      settings: SourceProductName=Simscape Electrical  SourceProductBaseCode=PS
  RMS : dspstat3/RMS  run=off  directionMode=Each column  dimension=1  InputProcessing=Columns as channels (frame based)  reset_popup=None
  Rate Transition : RateTransition  Integrity=off  Deterministic=off  OutPortSampleTime=100e-6
  Rate Transition1 : RateTransition  Integrity=off  Deterministic=off  OutPortSampleTime=100e-6
  Sum of Elements : Sum  Inputs=+
  Terminator : Terminator
  Terminator1 : Terminator
  Terminator2 : Terminator
  Unbuffer : Unbuffer
  Unbuffer1 : Unbuffer
  Load Power : Outport  VectorParamsAs1DForOutWhenUnconnected=off
  wires:
  Load shedding/1(Load Power) -> Load Power/1
  Vabc/1 -> Demux/1
  "[P0,Q0]"/1 -> Load shedding/3(load)
  Buffer1/1 -> RMS/1
  RMS/1 -> Unbuffer/1
  PLL/2 -> Terminator/1
  Unbuffer/1 -> Load shedding/2(Vamp_rms)
  Demux/3 -> Terminator1/1
  Demux/2 -> Terminator2/1
  Demux/1 -> Rate Transition1/1, Rate Transition/1
  PLL/1 -> Buffer2/1
  Buffer2/1 -> Sum of Elements/1
  Sum of Elements/1 -> Gain/1
  Gain/1 -> Unbuffer1/1
  Unbuffer1/1 -> Load shedding/1(" f_PLL")
  Rate Transition/1 -> Buffer1/1
  Rate Transition1/1 -> PLL/1

== system IEEE5BusSystemModel_std_UFLS/Dynamic Load1/Load 8 ==
  note: 200ms buffer for average voltag and frequency
      | to avoid oscillation
  Vabc : Inport
  "[P0,Q0]" : Inport  Port=2
  Buffer1 : Buffer  N=2400  V=2200
  Buffer2 : Buffer  N=240  V=220
  Demux : Demux  Outputs=[1 1 1]
  Gain : Gain  Gain=1/240
  Load shedding : Subsystem  TreatAsAtomicUnit=on  SystemSampleTime=20e-3
  PLL : powerlib_meascontrol/PLL/PLL  Fmin=45  Par_Init=[0, 50]  ParK=[180, 3200, 1]  TcD=1e-3  MaxRateChangeFreq=25  FilterCutOffFreq=25  Ts=1000e-6  AGC=on
      settings: SourceProductName=Simscape Electrical  SourceProductBaseCode=PS
  RMS : dspstat3/RMS  run=off  directionMode=Each column  dimension=1  InputProcessing=Columns as channels (frame based)  reset_popup=None
  Rate Transition : RateTransition  Integrity=off  Deterministic=off  OutPortSampleTime=100e-6
  Rate Transition1 : RateTransition  Integrity=off  Deterministic=off  OutPortSampleTime=100e-6
  Sum of Elements : Sum  Inputs=+
  Terminator : Terminator
  Terminator1 : Terminator
  Terminator2 : Terminator
  Unbuffer : Unbuffer
  Unbuffer1 : Unbuffer
  Load Power : Outport  VectorParamsAs1DForOutWhenUnconnected=off
  wires:
  Rate Transition1/1 -> PLL/1
  Rate Transition/1 -> Buffer1/1
  Unbuffer1/1 -> Load shedding/1(" f_PLL")
  Gain/1 -> Unbuffer1/1
  Sum of Elements/1 -> Gain/1
  Buffer2/1 -> Sum of Elements/1
  PLL/1 -> Buffer2/1
  Demux/1 -> Rate Transition/1, Rate Transition1/1
  Demux/2 -> Terminator2/1
  Demux/3 -> Terminator1/1
  Unbuffer/1 -> Load shedding/2(Vamp_rms)
  PLL/2 -> Terminator/1
  RMS/1 -> Unbuffer/1
  Buffer1/1 -> RMS/1
  "[P0,Q0]"/1 -> Load shedding/3(load)
  Vabc/1 -> Demux/1
  Load shedding/1(Load Power) -> Load Power/1

== system IEEE5BusSystemModel_std_UFLS/Dynamic Load2/Load 8 ==
  note: 200ms buffer for average voltag and frequency
      | to avoid oscillation
  Vabc : Inport
  "[P0,Q0]" : Inport  Port=2
  Buffer1 : Buffer  N=2400  V=2200
  Buffer2 : Buffer  N=240  V=220
  Demux : Demux  Outputs=[1 1 1]
  Gain : Gain  Gain=1/240
  Load shedding : Subsystem  TreatAsAtomicUnit=on  SystemSampleTime=20e-3
  PLL : powerlib_meascontrol/PLL/PLL  Fmin=45  Par_Init=[0, 50]  ParK=[180, 3200, 1]  TcD=1e-3  MaxRateChangeFreq=25  FilterCutOffFreq=25  Ts=1000e-6  AGC=on
      settings: SourceProductName=Simscape Electrical  SourceProductBaseCode=PS
  RMS : dspstat3/RMS  run=off  directionMode=Each column  dimension=1  InputProcessing=Columns as channels (frame based)  reset_popup=None
  Rate Transition : RateTransition  Integrity=off  Deterministic=off  OutPortSampleTime=100e-6
  Rate Transition1 : RateTransition  Integrity=off  Deterministic=off  OutPortSampleTime=100e-6
  Sum of Elements : Sum  Inputs=+
  Terminator : Terminator
  Terminator1 : Terminator
  Terminator2 : Terminator
  Unbuffer : Unbuffer
  Unbuffer1 : Unbuffer
  Load Power : Outport  VectorParamsAs1DForOutWhenUnconnected=off
  wires:
  Load shedding/1(Load Power) -> Load Power/1
  Vabc/1 -> Demux/1
  "[P0,Q0]"/1 -> Load shedding/3(load)
  Buffer1/1 -> RMS/1
  RMS/1 -> Unbuffer/1
  PLL/2 -> Terminator/1
  Unbuffer/1 -> Load shedding/2(Vamp_rms)
  Demux/3 -> Terminator1/1
  Demux/2 -> Terminator2/1
  Demux/1 -> Rate Transition1/1, Rate Transition/1
  PLL/1 -> Buffer2/1
  Buffer2/1 -> Sum of Elements/1
  Sum of Elements/1 -> Gain/1
  Gain/1 -> Unbuffer1/1
  Unbuffer1/1 -> Load shedding/1(" f_PLL")
  Rate Transition/1 -> Buffer1/1
  Rate Transition1/1 -> PLL/1

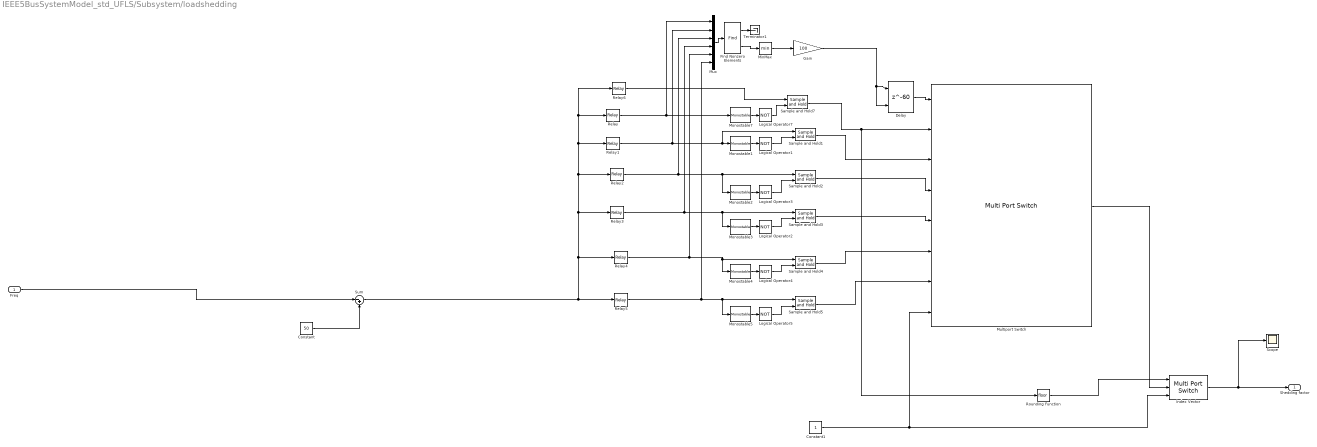
== system IEEE5BusSystemModel_std_UFLS/Subsystem/loadshedding ==
  Freq : Inport
  Constant : Constant  Value=50
  Constant1 : Constant
  Delay : Delay  DelayLength=60  InitialCondition=100  ExternalReset=Falling
      settings: InputPortMap=u0,r5
  Find Nonzero Elements : Find  NumberOfInputDimensions=3  ShowOutputForNonzeroInputValues=on
  Gain : Gain  Gain=100
  Index Vector : MultiPortSwitch  DataPortOrder=Zero-based contiguous  Inputs=2  zeroidx=on
  Logical Operator{1..5,7} (6 alike) : Logic  Operator=NOT  AllPortsSameDT=off  OutDataTypeStr=boolean
  MinMax : MinMax
  Monostable{1..5,7} (6 alike) : powerlib_meascontrol/Logic/Monostable  EdgeDetect=Either  PulseDuration=0.15  ic=0  Ts=0.0025
      settings: SourceProductName=Simscape Electrical  SourceProductBaseCode=PS
  Multiport Switch : MultiPortSwitch  DataPortOrder=Specify indices  DataPortIndices={95,85,75,65,55,50,100}
  Mux : Mux  Inputs=6
  Relay : Relay  OnSwitchValue=1  OffSwitchValue=-100  OnOutputValue=0.95  OffOutputValue=1
  Relay1 : Relay  OnSwitchValue=1.2  OffSwitchValue=-100  OnOutputValue=0.85
  Relay2 : Relay  OnSwitchValue=1.4  OffSwitchValue=-100  OnOutputValue=0.75
  Relay3 : Relay  OnSwitchValue=1.6  OffSwitchValue=-100  OnOutputValue=0.65
  Relay4 : Relay  OnSwitchValue=1.8  OffSwitchValue=-100  OnOutputValue=0.55
  Relay5 : Relay  OnSwitchValue=2  OffSwitchValue=-100  OnOutputValue=0.5
  Relay6 : Relay  OnSwitchValue=1  OffSwitchValue=-100  OnOutputValue=0.95  OffOutputValue=1
  Rounding Function : Rounding
  Sample and Hold1 : powerlib_meascontrol/Additional Components/Sample and Hold  ic=0.95  Ts=0.0025
      settings: SourceProductName=Simscape Electrical  SourceProductBaseCode=PS
  Sample and Hold2 : powerlib_meascontrol/Additional Components/Sample and Hold  ic=0.85  Ts=0.0025
      settings: SourceProductName=Simscape Electrical  SourceProductBaseCode=PS
  Sample and Hold3 : powerlib_meascontrol/Additional Components/Sample and Hold  ic=0.75  Ts=0.0025
      settings: SourceProductName=Simscape Electrical  SourceProductBaseCode=PS
  Sample and Hold4 : powerlib_meascontrol/Additional Components/Sample and Hold  ic=0.65  Ts=0.0025
      settings: SourceProductName=Simscape Electrical  SourceProductBaseCode=PS
  Sample and Hold5 : powerlib_meascontrol/Additional Components/Sample and Hold  ic=0.55  Ts=0.0025
      settings: SourceProductName=Simscape Electrical  SourceProductBaseCode=PS
  Sample and Hold7 : powerlib_meascontrol/Additional Components/Sample and Hold  ic=1  Ts=0.0025
      settings: SourceProductName=Simscape Electrical  SourceProductBaseCode=PS
  Scope : Scope
  Sum : Sum  Inputs=|-+
  Terminator1 : Terminator
  Shedding factor : Outport  VectorParamsAs1DForOutWhenUnconnected=off
  wires:
  Index Vector/1 -> Scope/1, Shedding factor/1
  Find Nonzero Elements/2 -> MinMax/1
  MinMax/1 -> Gain/1
  Constant1/1 -> Multiport Switch/8, Index Vector/3
  Constant/1 -> Sum/2
  Monostable1/1 -> Logical Operator1/1
  Sample and Hold1/1 -> Multiport Switch/3
  Logical Operator1/1 -> Sample and Hold1/2
  Sum/1 -> Relay/1, Relay6/1, Relay1/1, Relay2/1, Relay3/1, Relay4/1, Relay5/1
  Relay1/1 -> Mux/2, Sample and Hold1/1, Monostable1/1
  Find Nonzero Elements/1 -> Terminator1/1
  Relay/1 -> Mux/1, Monostable7/1
  Freq/1 -> Sum/1
  Multiport Switch/1 -> Index Vector/2
  Logical Operator7/1 -> Sample and Hold7/2
  Mux/1 -> Find Nonzero Elements/1
  Sample and Hold3/1 -> Multiport Switch/5
  Monostable7/1 -> Logical Operator7/1
  Sample and Hold2/1 -> Multiport Switch/4
  Relay2/1 -> Mux/3, Monostable2/1, Sample and Hold2/1
  Monostable2/1 -> Logical Operator3/1
  Logical Operator3/1 -> Sample and Hold2/2
  Monostable5/1 -> Logical Operator5/1
  Logical Operator2/1 -> Sample and Hold3/2
  Monostable3/1 -> Logical Operator2/1
  Relay3/1 -> Mux/4, Monostable3/1, Sample and Hold3/1
  Monostable4/1 -> Logical Operator4/1
  Sample and Hold4/1 -> Multiport Switch/6
  Relay4/1 -> Mux/5, Sample and Hold4/1, Monostable4/1
  Logical Operator4/1 -> Sample and Hold4/2
  Relay5/1 -> Mux/6, Monostable5/1, Sample and Hold5/1
  Logical Operator5/1 -> Sample and Hold5/2
  Sample and Hold5/1 -> Multiport Switch/7
  Gain/1 -> Delay/2, Delay/1
  Rounding Function/1 -> Index Vector/1
  Delay/1 -> Multiport Switch/1
  Relay6/1 -> Sample and Hold7/1
  Sample and Hold7/1 -> Rounding Function/1, Multiport Switch/2

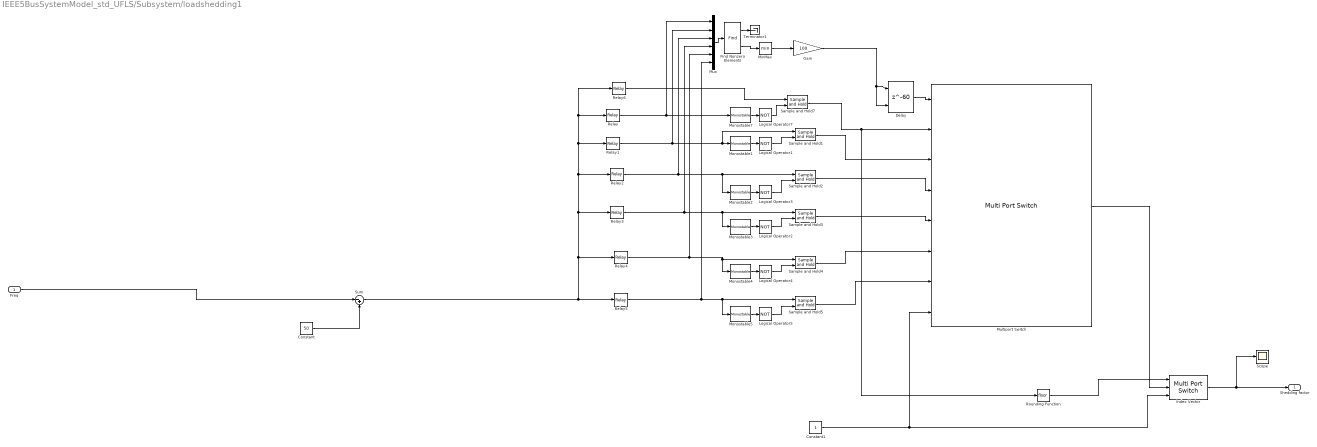
== system IEEE5BusSystemModel_std_UFLS/Subsystem/loadshedding1 ==
  Freq : Inport
  Constant : Constant  Value=50
  Constant1 : Constant
  Delay : Delay  DelayLength=60  InitialCondition=100  ExternalReset=Falling
      settings: InputPortMap=u0,r5
  Find Nonzero Elements : Find  NumberOfInputDimensions=3  ShowOutputForNonzeroInputValues=on
  Gain : Gain  Gain=100
  Index Vector : MultiPortSwitch  DataPortOrder=Zero-based contiguous  Inputs=2  zeroidx=on
  Logical Operator{1..5,7} (6 alike) : Logic  Operator=NOT  AllPortsSameDT=off  OutDataTypeStr=boolean
  MinMax : MinMax
  Monostable{1..5,7} (6 alike) : powerlib_meascontrol/Logic/Monostable  EdgeDetect=Either  PulseDuration=0.15  ic=0  Ts=0.0025
      settings: SourceProductName=Simscape Electrical  SourceProductBaseCode=PS
  Multiport Switch : MultiPortSwitch  DataPortOrder=Specify indices  DataPortIndices={95,85,75,65,55,50,100}
  Mux : Mux  Inputs=6
  Relay : Relay  OnSwitchValue=1  OffSwitchValue=-100  OnOutputValue=0.95  OffOutputValue=1
  Relay1 : Relay  OnSwitchValue=1.2  OffSwitchValue=-100  OnOutputValue=0.85
  Relay2 : Relay  OnSwitchValue=1.4  OffSwitchValue=-100  OnOutputValue=0.75
  Relay3 : Relay  OnSwitchValue=1.6  OffSwitchValue=-100  OnOutputValue=0.65
  Relay4 : Relay  OnSwitchValue=1.8  OffSwitchValue=-100  OnOutputValue=0.55
  Relay5 : Relay  OnSwitchValue=2  OffSwitchValue=-100  OnOutputValue=0.5
  Relay6 : Relay  OnSwitchValue=1  OffSwitchValue=-100  OnOutputValue=0.95  OffOutputValue=1
  Rounding Function : Rounding
  Sample and Hold1 : powerlib_meascontrol/Additional Components/Sample and Hold  ic=0.95  Ts=0.0025
      settings: SourceProductName=Simscape Electrical  SourceProductBaseCode=PS
  Sample and Hold2 : powerlib_meascontrol/Additional Components/Sample and Hold  ic=0.85  Ts=0.0025
      settings: SourceProductName=Simscape Electrical  SourceProductBaseCode=PS
  Sample and Hold3 : powerlib_meascontrol/Additional Components/Sample and Hold  ic=0.75  Ts=0.0025
      settings: SourceProductName=Simscape Electrical  SourceProductBaseCode=PS
  Sample and Hold4 : powerlib_meascontrol/Additional Components/Sample and Hold  ic=0.65  Ts=0.0025
      settings: SourceProductName=Simscape Electrical  SourceProductBaseCode=PS
  Sample and Hold5 : powerlib_meascontrol/Additional Components/Sample and Hold  ic=0.55  Ts=0.0025
      settings: SourceProductName=Simscape Electrical  SourceProductBaseCode=PS
  Sample and Hold7 : powerlib_meascontrol/Additional Components/Sample and Hold  ic=1  Ts=0.0025
      settings: SourceProductName=Simscape Electrical  SourceProductBaseCode=PS
  Scope : Scope
  Sum : Sum  Inputs=|-+
  Terminator1 : Terminator
  Shedding factor : Outport  VectorParamsAs1DForOutWhenUnconnected=off
  wires:
  Sample and Hold7/1 -> Multiport Switch/2, Rounding Function/1
  Relay6/1 -> Sample and Hold7/1
  Delay/1 -> Multiport Switch/1
  Rounding Function/1 -> Index Vector/1
  Gain/1 -> Delay/1, Delay/2
  Sample and Hold5/1 -> Multiport Switch/7
  Logical Operator5/1 -> Sample and Hold5/2
  Relay5/1 -> Sample and Hold5/1, Monostable5/1, Mux/6
  Logical Operator4/1 -> Sample and Hold4/2
  Relay4/1 -> Monostable4/1, Sample and Hold4/1, Mux/5
  Sample and Hold4/1 -> Multiport Switch/6
  Monostable4/1 -> Logical Operator4/1
  Relay3/1 -> Sample and Hold3/1, Monostable3/1, Mux/4
  Monostable3/1 -> Logical Operator2/1
  Logical Operator2/1 -> Sample and Hold3/2
  Monostable5/1 -> Logical Operator5/1
  Logical Operator3/1 -> Sample and Hold2/2
  Monostable2/1 -> Logical Operator3/1
  Relay2/1 -> Sample and Hold2/1, Monostable2/1, Mux/3
  Sample and Hold2/1 -> Multiport Switch/4
  Monostable7/1 -> Logical Operator7/1
  Sample and Hold3/1 -> Multiport Switch/5
  Mux/1 -> Find Nonzero Elements/1
  Logical Operator7/1 -> Sample and Hold7/2
  Multiport Switch/1 -> Index Vector/2
  Freq/1 -> Sum/1
  Relay/1 -> Monostable7/1, Mux/1
  Find Nonzero Elements/1 -> Terminator1/1
  Relay1/1 -> Monostable1/1, Sample and Hold1/1, Mux/2
  Sum/1 -> Relay5/1, Relay4/1, Relay3/1, Relay2/1, Relay1/1, Relay6/1, Relay/1
  Logical Operator1/1 -> Sample and Hold1/2
  Sample and Hold1/1 -> Multiport Switch/3
  Monostable1/1 -> Logical Operator1/1
  Constant/1 -> Sum/2
  Constant1/1 -> Index Vector/3, Multiport Switch/8
  MinMax/1 -> Gain/1
  Find Nonzero Elements/2 -> MinMax/1
  Index Vector/1 -> Scope/1, Shedding factor/1

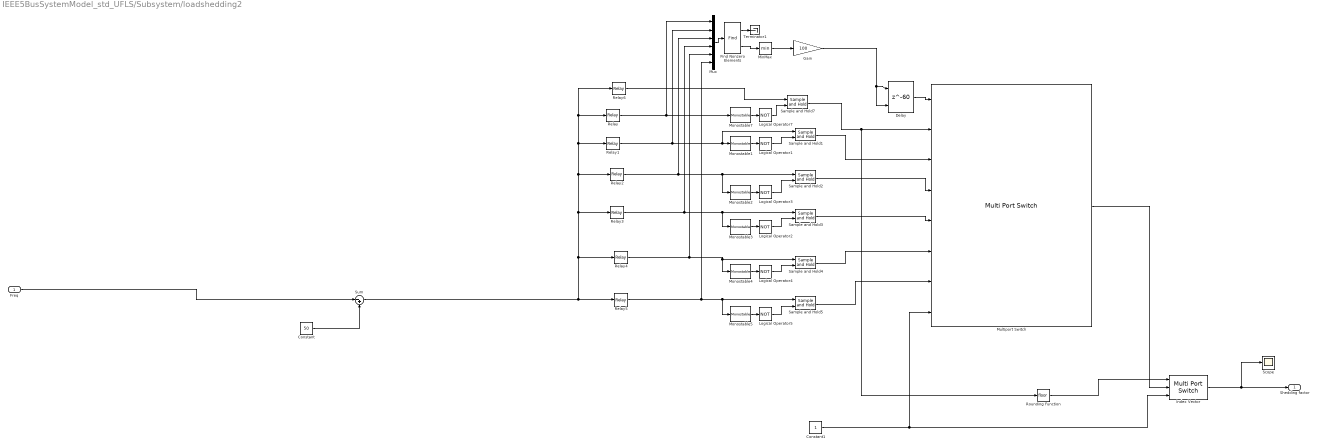
== system IEEE5BusSystemModel_std_UFLS/Subsystem/loadshedding2 ==
  Freq : Inport
  Constant : Constant  Value=50
  Constant1 : Constant
  Delay : Delay  DelayLength=60  InitialCondition=100  ExternalReset=Falling
      settings: InputPortMap=u0,r5
  Find Nonzero Elements : Find  NumberOfInputDimensions=3  ShowOutputForNonzeroInputValues=on
  Gain : Gain  Gain=100
  Index Vector : MultiPortSwitch  DataPortOrder=Zero-based contiguous  Inputs=2  zeroidx=on
  Logical Operator{1..5,7} (6 alike) : Logic  Operator=NOT  AllPortsSameDT=off  OutDataTypeStr=boolean
  MinMax : MinMax
  Monostable{1..5,7} (6 alike) : powerlib_meascontrol/Logic/Monostable  EdgeDetect=Either  PulseDuration=0.15  ic=0  Ts=0.0025
      settings: SourceProductName=Simscape Electrical  SourceProductBaseCode=PS
  Multiport Switch : MultiPortSwitch  DataPortOrder=Specify indices  DataPortIndices={95,85,75,65,55,50,100}
  Mux : Mux  Inputs=6
  Relay : Relay  OnSwitchValue=1  OffSwitchValue=-100  OnOutputValue=0.95  OffOutputValue=1
  Relay1 : Relay  OnSwitchValue=1.2  OffSwitchValue=-100  OnOutputValue=0.85
  Relay2 : Relay  OnSwitchValue=1.4  OffSwitchValue=-100  OnOutputValue=0.75
  Relay3 : Relay  OnSwitchValue=1.6  OffSwitchValue=-100  OnOutputValue=0.65
  Relay4 : Relay  OnSwitchValue=1.8  OffSwitchValue=-100  OnOutputValue=0.55
  Relay5 : Relay  OnSwitchValue=2  OffSwitchValue=-100  OnOutputValue=0.5
  Relay6 : Relay  OnSwitchValue=1  OffSwitchValue=-100  OnOutputValue=0.95  OffOutputValue=1
  Rounding Function : Rounding
  Sample and Hold1 : powerlib_meascontrol/Additional Components/Sample and Hold  ic=0.95  Ts=0.0025
      settings: SourceProductName=Simscape Electrical  SourceProductBaseCode=PS
  Sample and Hold2 : powerlib_meascontrol/Additional Components/Sample and Hold  ic=0.85  Ts=0.0025
      settings: SourceProductName=Simscape Electrical  SourceProductBaseCode=PS
  Sample and Hold3 : powerlib_meascontrol/Additional Components/Sample and Hold  ic=0.75  Ts=0.0025
      settings: SourceProductName=Simscape Electrical  SourceProductBaseCode=PS
  Sample and Hold4 : powerlib_meascontrol/Additional Components/Sample and Hold  ic=0.65  Ts=0.0025
      settings: SourceProductName=Simscape Electrical  SourceProductBaseCode=PS
  Sample and Hold5 : powerlib_meascontrol/Additional Components/Sample and Hold  ic=0.55  Ts=0.0025
      settings: SourceProductName=Simscape Electrical  SourceProductBaseCode=PS
  Sample and Hold7 : powerlib_meascontrol/Additional Components/Sample and Hold  ic=1  Ts=0.0025
      settings: SourceProductName=Simscape Electrical  SourceProductBaseCode=PS
  Scope : Scope
  Sum : Sum  Inputs=|-+
  Terminator1 : Terminator
  Shedding factor : Outport  VectorParamsAs1DForOutWhenUnconnected=off
  wires:
  Index Vector/1 -> Scope/1, Shedding factor/1
  Find Nonzero Elements/2 -> MinMax/1
  MinMax/1 -> Gain/1
  Constant1/1 -> Multiport Switch/8, Index Vector/3
  Constant/1 -> Sum/2
  Monostable1/1 -> Logical Operator1/1
  Sample and Hold1/1 -> Multiport Switch/3
  Logical Operator1/1 -> Sample and Hold1/2
  Sum/1 -> Relay/1, Relay6/1, Relay1/1, Relay2/1, Relay3/1, Relay4/1, Relay5/1
  Relay1/1 -> Mux/2, Sample and Hold1/1, Monostable1/1
  Find Nonzero Elements/1 -> Terminator1/1
  Relay/1 -> Mux/1, Monostable7/1
  Freq/1 -> Sum/1
  Multiport Switch/1 -> Index Vector/2
  Logical Operator7/1 -> Sample and Hold7/2
  Mux/1 -> Find Nonzero Elements/1
  Sample and Hold3/1 -> Multiport Switch/5
  Monostable7/1 -> Logical Operator7/1
  Sample and Hold2/1 -> Multiport Switch/4
  Relay2/1 -> Mux/3, Monostable2/1, Sample and Hold2/1
  Monostable2/1 -> Logical Operator3/1
  Logical Operator3/1 -> Sample and Hold2/2
  Monostable5/1 -> Logical Operator5/1
  Logical Operator2/1 -> Sample and Hold3/2
  Monostable3/1 -> Logical Operator2/1
  Relay3/1 -> Mux/4, Monostable3/1, Sample and Hold3/1
  Monostable4/1 -> Logical Operator4/1
  Sample and Hold4/1 -> Multiport Switch/6
  Relay4/1 -> Mux/5, Sample and Hold4/1, Monostable4/1
  Logical Operator4/1 -> Sample and Hold4/2
  Relay5/1 -> Mux/6, Monostable5/1, Sample and Hold5/1
  Logical Operator5/1 -> Sample and Hold5/2
  Sample and Hold5/1 -> Multiport Switch/7
  Gain/1 -> Delay/2, Delay/1
  Rounding Function/1 -> Index Vector/1
  Delay/1 -> Multiport Switch/1
  Relay6/1 -> Sample and Hold7/1
  Sample and Hold7/1 -> Rounding Function/1, Multiport Switch/2

== system IEEE5BusSystemModel_std_UFLS/Subsystem1/PMU_e-IpDFT_P-class ==
  Uabc : Inport
  Constant1 : Constant  Value=dF  SampleTime=Ts_p
  Constant2 : Constant  Value=0  SampleTime=Ts_p
  Counter : dspswit3/Counter  Direction=Up  CountEvent=Free running  CounterSize=User defined  MaxCount=M-1  InitialCount=1  Output=Hit  HitValue=0  ResetInput=off  SamplesPerFrame=1  Ts=Ts_p  CntDtype=double  HitDtype=Logical
  Demux1 : Demux  Outputs=3
  Ia_est : Subsystem
  Terminator3 : Terminator
  Terminator4 : Terminator
  Frequency : Outport  VectorParamsAs1DForOutWhenUnconnected=off
  Amplitude : Outport  Port=2  VectorParamsAs1DForOutWhenUnconnected=off
  Phase : Outport  Port=3  VectorParamsAs1DForOutWhenUnconnected=off
  wires:
  Demux1/3 -> Terminator4/1
  Demux1/2 -> Terminator3/1
  Constant2/1 -> Ia_est/3(dT [s])
  Constant1/1 -> Ia_est/4(dF [Hz])
  Counter/1 -> Ia_est/2(Hit)
  Demux1/1 -> Ia_est/1(signal)
  Uabc/1 -> Demux1/1
  Ia_est/3(Phase) -> Phase/1
  Ia_est/2(Amplitude) -> Amplitude/1
  Ia_est/1(Frequency) -> Frequency/1

== system IEEE5BusSystemModel_std_UFLS/Subsystem1/PMU_e-IpDFT_P-class1 ==
  Uabc : Inport
  Constant1 : Constant  Value=dF  SampleTime=Ts_p
  Constant2 : Constant  Value=0  SampleTime=Ts_p
  Counter : dspswit3/Counter  Direction=Up  CountEvent=Free running  CounterSize=User defined  MaxCount=M-1  InitialCount=1  Output=Hit  HitValue=0  ResetInput=off  SamplesPerFrame=1  Ts=Ts_p  CntDtype=double  HitDtype=Logical
  Demux1 : Demux  Outputs=3
  Ia_est : Subsystem
  Terminator3 : Terminator
  Terminator4 : Terminator
  Frequency : Outport  VectorParamsAs1DForOutWhenUnconnected=off
  Amplitude : Outport  Port=2  VectorParamsAs1DForOutWhenUnconnected=off
  Phase : Outport  Port=3  VectorParamsAs1DForOutWhenUnconnected=off
  wires:
  Ia_est/1(Frequency) -> Frequency/1
  Ia_est/2(Amplitude) -> Amplitude/1
  Ia_est/3(Phase) -> Phase/1
  Uabc/1 -> Demux1/1
  Demux1/1 -> Ia_est/1(signal)
  Counter/1 -> Ia_est/2(Hit)
  Constant1/1 -> Ia_est/4(dF [Hz])
  Constant2/1 -> Ia_est/3(dT [s])
  Demux1/2 -> Terminator3/1
  Demux1/3 -> Terminator4/1
